simulink model "Longitudinal_old"  (R2025b)
settings: Solver=VariableStepAuto  StartTime=0.0  StopTime=100  RelTol=1e-3
undefined symbols (not defined in the file): car, m, R, Tau_1, Tau_2, Tau_3, Tau_4, Tau_EM, tyre
libraries: simulink x4
(part 2 of 2)

== matlab function Longitudinal_old/longitudinal dynamics/Min Fx solver/FR ==
  data: Fx_EM input; Fx_FR output; Fx_tyre input; delta_Fx_FR output
function [Fx_FR, delta_Fx_FR] = fcn(Fx_EM, Fx_tyre)

% add delta Fx for each tyre

if Fx_EM<Fx_tire
    Fx_FR = Fx_EM;
else 
    Fx_FR = Fx_tire;
    delta_Fx_FR = Fx_EM - Fx_tire;
end

== matlab function Longitudinal_old/longitudinal dynamics/Min Fx solver/FL ==
  data: Fx_EM input; Fx_FL output; Fx_tyre input; delta_Fx_FL output
function [Fx_FL, delta_Fx_FL] = fcn(Fx_EM, Fx_tyre)

% add delta Fx for each tyre

if Fx_EM<Fx_tire
    Fx_FL = Fx_EM;
else 
    Fx_FL = Fx_tire;
    delta_Fx_FL = Fx_EM - Fx_tire;
end

== matlab function Longitudinal_old/Powertrain/Driver model - gear selection/MATLAB Function3 ==
  settings: updateMethod=CONTINUOUS
  data: w_ICE input; gear_trigger output; gear_in input; gear_out output
function [gear_trigger, gear_out] = change_gear(w_ICE, gear_in)

% --- Parametri ---
R = 0.203;                                  % raggio ruota [m]
gear_trigger = 0;
v = w_ICE*R;
v_thresh = [89.8, 102.4];                    % soglie cambio
tau = [2.785, 2.052, 1.714, 1.5];           % rapporti di trasmissione

if gear_in >= numel(tau) || v < v_thresh(gear_in)
    return
    
elseif v >= v_thresh(gear_in) && gear_trigger == 0
    gear_in = gear_in + 1;                    % cambia marcia
    gear_trigger = 1;
    gear_out = gear_in;
end

== matlab function Longitudinal_old/longitudinal dynamics/Subsystem/FL ==
  data: delta_Fx_front input; delta_z_tyre input; w_dot_tyre_FL output
function w_dot_tyre_FL  = fcn(delta_Fx_front, delta_z_tyre)

w_dot_tyre_front = delta_Fx_front * (R - delta_z_tyre_front) * eta_pwt / J_f;

== matlab function Longitudinal_old/longitudinal dynamics/Subsystem/RL ==
  data: delta_Fx_rear input; w_dot_tyre_RL output; delta_z_tyre input
function w_dot_tyre_RL  = fcn(delta_Fx_rear, delta_z_tyre)

% use bus for all tyres

w_dot_tyre_rear = delta_Fx_rear * (R - delta_z_tyre_rear) * eta_pwt / J_r;

== matlab function Longitudinal_old/longitudinal dynamics/Fx equilibrium ==
  data: Fz_FL output; a input; Fz_RR output; Fz_RL output; Fz_FR output; delta_Fz output; v input; Drag output; Cx input; Cz input
function [Fz_FL, Fz_RR, Fz_RL, Fz_FR, delta_Fz, Drag] = fx_equilibrium(a, v,Cx,Cz)

Downforce = 0.5 * rho * Cz * A * v ^ 2; % downforce
Drag = 0.5 * rho * Cx * A * v ^2; % drag
M_aero = Drag * (h_cp - h_cog) - Downforce * (lf-x_cp);

delta_Fz = m * a * h_cog / wb + Drag * h_cog / wb + M_aero / wb;

Fz_front = -(m * a + Drag) * h_cog / wb + ( m * g - Downforce ) * (lr -delta) / wb - M_aero / wb - J_f * a / (R * wb);

Fz_FR = Fz_front / 2;
Fz_FL = Fz_FR;

Fz_rear = (m * a + Drag) * h_cog / wb + ( m * g - Downforce ) * (lf + delta) / wb + M_aero / wb + J_r * a / (R * wb);

Fz_RR = Fz_rear / 2;
Fz_RL = Fz_RR;

== matlab function Longitudinal_old/longitudinal dynamics/Fx powertrain calculation/FL ==
  data: Fz input; Fx_EM_FL output; T input
function Fx_EM_FL = fcn(Fz, T)

Fx_EM_FL = (T - Fz * delta - J_f * a / R) / R ; % J - parameter for each tyre - J_f & J_r

== matlab function Longitudinal_old/Tyres/Rear Right ==
  data: tyre input; Fx_RR output; SR input; Fz input; camber input
function Fx_RR = fcn(tyre,SR,Fz,camber)

% PAC2002 puro longitudinale (Fx vs k)

     Fz0 = tyre.Fz0;
     if Fz0 == 0, Fz0 = max(1, Fz); end
    dfz = (Fz - Fz0)/Fz0;

    pi0 = tyre.pi0;  % Pa nominale
    dpi = (tyre.pressure.rear - pi0)/pi0;
    
    Cx1 = tyre.Cx1;
    Dx1 = tyre.Dx1;
    Dx2 = tyre.Dx2;
    Dx3 = tyre.Dx3;
    Ex1 = tyre.Ex1;
    Ex2 = tyre.Ex2;
    Ex3 = tyre.Ex3;
    Ex4 = tyre.Ex4;
    Kx1 = tyre.Kx1;
    Kx2 = tyre.Kx2;
    Kx3 = tyre.Kx3;
    Hx1 = tyre.Hx1;
    Hx2 = tyre.Hx2;
    Vx1 = tyre.Vx1;
    Vx2 = tyre.Vx2;
    px1 = tyre.px1;
    px2 = tyre.px2;
    px3 = tyre.px3;
    px4 = tyre.px4;
    lmux = tyre.lmux;

    gamma = camber*pi/180;
    mu = (Dx1 + Dx2*dfz) * (1 - Dx3*(gamma^2)) * (1 + px3*dpi + px4*dpi^2)*lmux;
    % mu = 1.4;

    D = mu * Fz;
    C = Cx1;
    K = Fz * (Kx1 + Kx2*dfz) * exp(Kx3*dfz) * (1 + px1*dpi + px2*dpi^2);
    B = K / (C*D + eps);

    SH = Hx1 + Hx2*dfz;
    SR  = SR + SH;

    E  = (Ex1 + Ex2*dfz + Ex3*dfz^2) * (1 - Ex4*sign(SR));
    SV = Fz * (Vx1 + Vx2*dfz);

    Fx0 = D * sin( C * atan( B*SR - E*(B*SR - atan(B*SR)) ) );
    Fx_RR = Fx0 + SV;

== matlab function Longitudinal_old/Tyres/Front Right ==
  data: tyre input; SR input; Fx_FR output; Fz input; camber input
function Fx_FR = fcn(tyre,SR,Fz,camber)

% PAC2002 puro longitudinale (Fx vs k)

     Fz0 = tyre.Fz0;
     if Fz0 == 0, Fz0 = max(1, Fz); end
    dfz = (Fz - Fz0)/Fz0;

    pi0 = tyre.pi0;  % Pa nominale
    dpi = (tyre.pressure.front - pi0)/pi0;
    
    Cx1 = tyre.Cx1;
    Dx1 = tyre.Dx1;
    Dx2 = tyre.Dx2;
    Dx3 = tyre.Dx3;
    Ex1 = tyre.Ex1;
    Ex2 = tyre.Ex2;
    Ex3 = tyre.Ex3;
    Ex4 = tyre.Ex4;
    Kx1 = tyre.Kx1;
    Kx2 = tyre.Kx2;
    Kx3 = tyre.Kx3;
    Hx1 = tyre.Hx1;
    Hx2 = tyre.Hx2;
    Vx1 = tyre.Vx1;
    Vx2 = tyre.Vx2;
    px1 = tyre.px1;
    px2 = tyre.px2;
    px3 = tyre.px3;
    px4 = tyre.px4;
    lmux = tyre.lmux;

    gamma = camber*pi/180;
    mu = (Dx1 + Dx2*dfz) * (1 - Dx3*(gamma^2)) * (1 + px3*dpi + px4*dpi^2)*lmux;
    % mu = 1.4;

    D = mu * Fz;
    C = Cx1;
    K = Fz * (Kx1 + Kx2*dfz) * exp(Kx3*dfz) * (1 + px1*dpi + px2*dpi^2);
    B = K / (C*D + eps);

    SH = Hx1 + Hx2*dfz;
    SR  = SR + SH;

    E  = (Ex1 + Ex2*dfz + Ex3*dfz^2) * (1 - Ex4*sign(SR));
    SV = Fz * (Vx1 + Vx2*dfz);

    Fx0 = D * sin( C * atan( B*SR - E*(B*SR - atan(B*SR)) ) );
    Fx_FR = Fx0 + SV;

== matlab function Longitudinal_old/Tyres/Rear Left ==
  data: tyre input; Fx_RL output; SR input; Fz input; camber input
function Fx_RL = fcn(tyre,SR,Fz,camber)

% PAC2002 puro longitudinale (Fx vs k)

     Fz0 = tyre.Fz0;
     if Fz0 == 0, Fz0 = max(1, Fz); end
    dfz = (Fz - Fz0)/Fz0;

    pi0 = tyre.pi0;  % Pa nominale
    dpi = (tyre.pressure.rear - pi0)/pi0;
    
    Cx1 = tyre.Cx1;
    Dx1 = tyre.Dx1;
    Dx2 = tyre.Dx2;
    Dx3 = tyre.Dx3;
    Ex1 = tyre.Ex1;
    Ex2 = tyre.Ex2;
    Ex3 = tyre.Ex3;
    Ex4 = tyre.Ex4;
    Kx1 = tyre.Kx1;
    Kx2 = tyre.Kx2;
    Kx3 = tyre.Kx3;
    Hx1 = tyre.Hx1;
    Hx2 = tyre.Hx2;
    Vx1 = tyre.Vx1;
    Vx2 = tyre.Vx2;
    px1 = tyre.px1;
    px2 = tyre.px2;
    px3 = tyre.px3;
    px4 = tyre.px4;
    lmux = tyre.lmux;

    gamma = camber*pi/180;
    mu = (Dx1 + Dx2*dfz) * (1 - Dx3*(gamma^2)) * (1 + px3*dpi + px4*dpi^2)*lmux;
    % mu = 1.4;

    D = mu * Fz;
    C = Cx1;
    K = Fz * (Kx1 + Kx2*dfz) * exp(Kx3*dfz) * (1 + px1*dpi + px2*dpi^2);
    B = K / (C*D + eps);

    SH = Hx1 + Hx2*dfz;
    SR  = SR + SH;

    E  = (Ex1 + Ex2*dfz + Ex3*dfz^2) * (1 - Ex4*sign(SR));
    SV = Fz * (Vx1 + Vx2*dfz);

    Fx0 = D * sin( C * atan( B*SR - E*(B*SR - atan(B*SR)) ) );
    Fx_RL = Fx0 + SV;

== matlab function Longitudinal_old/longitudinal dynamics/Kinematics/RL/Rear tyre ==
  data: wheel_travel_RL output; IR input; AS input; AD input; h_ground output; Fz input; delta_Fz input; jounce_rear output
function [wheel_travel_RL, h_ground, jounce_rear]      = kinematics(IR, AS, AD, Fz, delta_Fz)

delta_z_tyre = Fz / kz_tyre; % tyre vertical stiffness - kz_tyre - for front and rear tyres, look at buses
k_spring_ground = (k_spring * IR^2);

if a > 0 % under acceleration
    delta_z_spring_rear = (Fz - delta_Fz) / k_spring_ground + delta_Fz * ((1-AS)/k_spring_ground) ; % rear axle
else % under braking
    delta_z_spring_rear = Fz / k_spring_ground; % rear axle
end

wheel_travel_rear = delta_z_spring_rear - z0_spring_rear; % if negative it is bounce

jounce_rear = delta_z_tyre + delta_z_spring_rear - z0_rear;

% h_ground_front = ;
% h_ground_rear = ;

% h_ground = delta_z - z_0;
% wheel_travel =  h_ground - delta_z_tyre;

% does the AS contribute to less tyre deflection or just smaller spring
% deflection?
% static height - how do we take it - when wheels are on the ground
